simulink model "state_equation_pendulum"  (R2024a)
settings: Solver=ode5  StartTime=0.0  StopTime=10.0  FixedStep=0.001  RelTol=1e-3
settings Model: Creator=ADMIN  LastModifiedBy=ADMIN

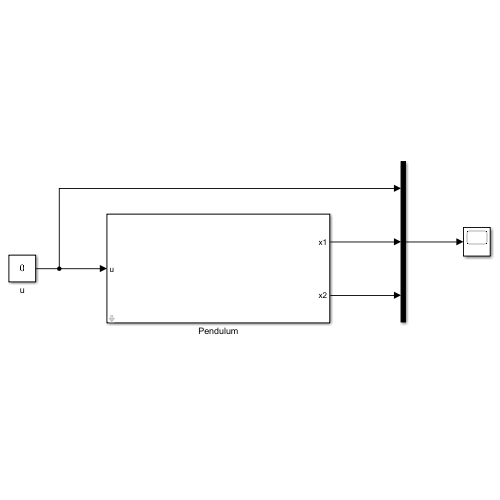
[thumbnail: Simulink's stored preview of the top-level diagram]
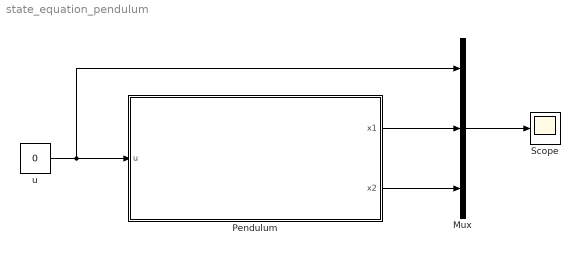
== system state_equation_pendulum ==
  Mux : Mux  Inputs=3
  Pendulum : Subsystem  mask{m=0, l=0, B=0, g=0, x1_init=0, x2_init=0}
      mask prompts: m "Pendulum Mass"; l "Pendulum Length"; B "Coeff of Friction"; g "Coeff of Gravity"; x1_init "Init Angle of the Pendulum"; x2_init "Init Vel of the Pendulum"
  Scope : Scope
  u : Constant  Value=0
  wires:
  u/1 -> Mux/1, Pendulum/1(u)
  Pendulum/1(x1) -> Mux/2
  Pendulum/2(x2) -> Mux/3
  Mux/1 -> Scope/1

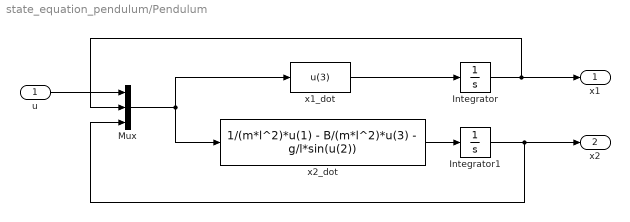
== system state_equation_pendulum/Pendulum ==
  u : Inport
  Integrator : Integrator  InitialCondition=x1_init
  Integrator1 : Integrator  InitialCondition=x2_init
  Mux : Mux  Inputs=3
  x1_dot : Fcn  Expr=u(3)
  x2_dot : Fcn  Expr=1/(m*l^2)*u(1) - B/(m*l^2)*u(3) - g/l*sin(u(2))
  x1 : Outport
  x2 : Outport  Port=2
  wires:
  Integrator1/1 -> x2/1, Mux/3
  u/1 -> Mux/1
  x1_dot/1 -> Integrator/1
  Mux/1 -> x2_dot/1, x1_dot/1
  Integrator/1 -> x1/1, Mux/2
  x2_dot/1 -> Integrator1/1
